simulink model "tire"  (R2017b)
settings: Solver=VariableStepAuto  StartTime=0.0  StopTime=30  RelTol=1e-3
libraries: simulink x1
settings Model: Creator=ashwin.ramanujam  LastModifiedBy=Vjekoslav

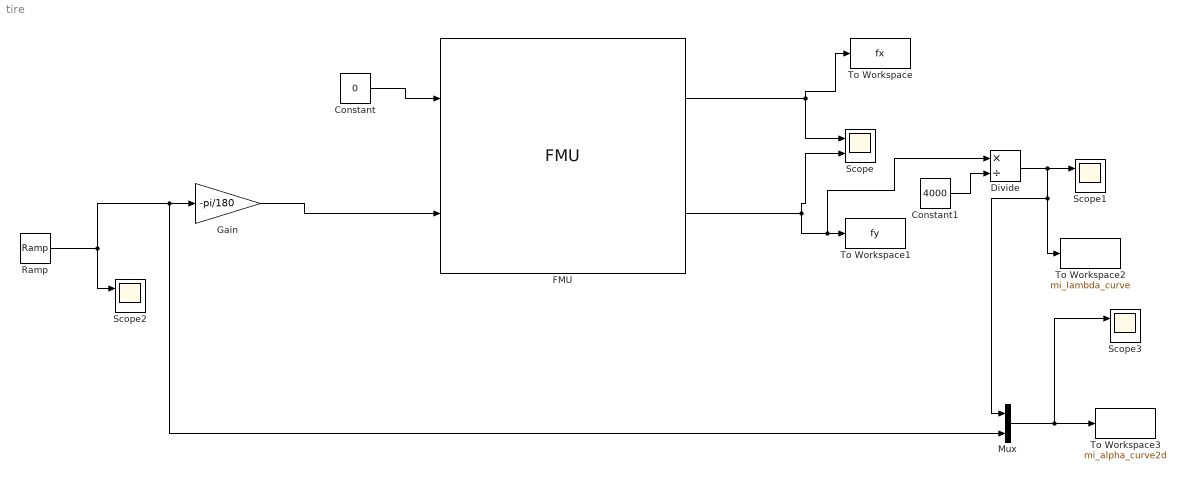
== system tire ==
  Constant : Constant  Value=0
  Constant1 : Constant  Value=4000
  Divide : Product  Inputs=*/
  FMU : FMU  FMUName=MED2018_TireTest.fmu  FMUMode=CoSimulation  wheel=struct('left_wheel',boolean(true),'wheel_number',int32(1),'m',10,'i_xx',1,'contact',struct('generic',struct('v_start',10)),'forces',struct('left_parameters',boolean(true),'verticalDynamics',struct('rho_transition',0.01),'inside_of_valid',struct('k',1)),'visualization',struct('rim2',struct('R0',0.3,'spoke_thickness',0.05)),'hub',struct('rev',struct('phi0',0,'stateSelect',int32(4)),'wheelBody',struct('rbr',[0,0,0],'rcm',[0,0,0],'R_cm',struct('T',reshape([1.0,0.0,0.0,0.0,1.0,0.0,0.0,0.0,1.0], [3,3]),'w',[0.0,0.0,0.0]),'i_21',0,'i_31',0,'i_32',0),'carrierForce',struct('N_to_m',1000),'carrierTorque',struct('Nm_to_m',1000)),'CZ',200000.0,'KZ',500.0,'FNOMIN',4100,'BREFF',8.4,'DREFF',0.27,'FREFF',0.07,'LFZ0',1,'LCX',1,'LMUX',1,'LEX',1,'LKX',1,'LHX',1,'LVX',1,'LGAX',1,'LCY',1,'LMUY',1,'LEY',1,'LKY',1,'LHY',1,'LVY',1,'LGAY',1,'LTR',1,'LRES',0,'LGAZ',1,'LMX',1,'LVMX',1,'LMY',1,'LXAL',1,'LYKA',1,'LVYKA',1,'LS',1,'LSGKP',1,'LSGAL',1,'LGYR',1,'PCX1',1.63,'PDX1',1.06,'PDX2',-0.0492,'PDX3',-2.29,'PEX1',0.5,'PEX2',-0.11,'PEX3',-0.06,'PEX4',0,'PKX1',19.7,'PKX2',-0.15,'PKX3',0.18,'PHX1',-0.0005,'PHX2',8.5E-05,'PVX1',0,'PVX2',0,'PCY1',1.28,'PDY1',-0.92,'PDY2',0.22,'PDY3',-4.55,'PEY1',-1.1,'PEY2',0.65,'PEY3',-0.65,'PEY4',-12.41,'PKY1',-13.06,'PKY2',1.77,'PKY3',0.19,'PHY1',0.0034,'PHY2',-0.003,'PHY3',0.044,'PVY1',0.044,'PVY2',-0.03,'PVY3',-0.176,'PVY4',-0.44,'QBZ1',8.4,'QBZ2',-2.96,'QBZ3',0.45,'QBZ4',-0.45,'QBZ5',-0.45,'QBZ9',3.45,'QBZ10',0,'QCZ1',1.2,'QDZ1',0.1,'QDZ2',-0.003,'QDZ3',-0.55,'QDZ4',8.4,'QDZ6',-0.003,'QDZ7',0.005,'QDZ8',-0.11,'QDZ9',0.11,'QEZ1',-2.9,'QEZ2',-0.5,'QEZ3',0,'QEZ4',-0.12,'QEZ5',-3.71,'QHZ1',0.003,'QHZ2',0.00084,'QHZ3',0.158,'QHZ4',0.121,'RBX1',9.0,'RBX2',-8.6,'RCX1',1.131,'REX1',0.081,'REX2',-0.15,'RHX1',-0.029,'RBY1',6.4,'RBY2',7.91,'RBY3',-0.059,'RCY1',1.16,'REY1',0.22,'REY2',0.43,'RHY1',0.0007,'RHY2',0.023,'RVY1',0,'RVY2',0,'RVY3',0,'RVY4',10,'RVY5',1.94,'RVY6',-50,'SSZ1',0.023,'SSZ2',0.019,'SSZ3',0.5,'SSZ4',-0.28,'QSX1',0.032,'QSX2',0.49,'QSX3',0.12,'QSY3',0,'QSY4',0,'LONGVL',16.5,'PTX1',1.98,'PTX2',0.0003,'PTX3',-0.31,'PTY1',1.8,'PTY2',1.8,'QTZ1',0.2,'MBELT',4.1)  rig=struct('xTranslation',struct('s0',0,'stateSelect',int32(4)),'yTranslation',struct('s0',0,'stateSelect',int32(4)),'zTranslation',struct('stateSelect',int32(4)),'xMotionEntity',struct('f_crit',50,'fixed_offset',boolean(true)),'yMotionEntity',struct('f_crit',50),'zMotionEntity',struct('f_crit',50),'steerMotionEntity',struct('f_crit',50),'camberMotionEntity',struct('f_crit',50),'steeringAngle',struct('phi0',0,'stateSelect',int32(4)),'camberAngle',struct('phi0',0,'stateSelect',int32(4)),'piston',struct('r1',[0,0,0],'r2',[0,0,0]),'hub',struct('f_crit',50,'fixed_offset',boolean(true),'actuator',struct('vel',struct('phi0',0))),'gain1',struct('k',-1))  setup=struct('gamma_deg',0,'sweep_time',10)  F_z=4000  V_x=16.7  FMUSampleTime=[0.001,0]  mask(MED2018.TireTest [Co-Simulation, v2.0]){}
      mask Display:
      | if (exist([Simulink.fileGenControl('get','CacheFolder') '\slprj\_fmu\2328b5e92424745d9fd7866ab0f1a964\MED2018_TireTest\model.png'],'file'))
      |     image([Simulink.fileGenControl('get','CacheFolder') '\slprj\_fmu\2328b5e92424745d9fd7866ab0f1a964\MED2018_TireTest\model.png']);
      |     text(0.03, 0.97, 'MED2018.TireTest', 'horizontalAlignment', 'left', 'verticalAlignment', 'top');
      | else
      |     disp('MED2018.TireTest');
      | end
      | port_label('output',1,'Fx');
      | port_label('output',2,'Fy');
      | port_label('input',1,'lambda');
      | port_label('input',2,'alpha');
  Gain : Gain  Gain=-pi/180
  Mux : Mux  Inputs=2
  Ramp : simulink/Sources/Ramp  slope=1  start=0  X0=-15
  Scope{,1..3} (4 alike) : Scope  NumInputPorts=2
  To Workspace : ToWorkspace  VariableName=fx  SaveFormat=Timeseries  SampleTime=-1
  To Workspace1 : ToWorkspace  VariableName=fy  SaveFormat=Timeseries  SampleTime=-1
  To Workspace2 : ToWorkspace  VariableName=mi_lambda_curve  SaveFormat=Timeseries  SampleTime=-1
  To Workspace3 : ToWorkspace  VariableName=mi_alpha_curve2d  SampleTime=-1
  wires:
  FMU/1 -> To Workspace/1, Scope/1
  FMU/2 -> Scope/2, Divide/1, To Workspace1/1
  Constant1/1 -> Divide/2
  Divide/1 -> Mux/1, To Workspace2/1, Scope1/1
  Gain/1 -> FMU/2
  Constant/1 -> FMU/1
  Mux/1 -> Scope3/1, To Workspace3/1
  Ramp/1 -> Scope2/1, Mux/2, Gain/1
